simulink model "prob1"  (R2020a)
settings: Solver=VariableStepAuto  StartTime=0.0  StopTime=50  RelTol=1e-3
model workspace (MAT data in the model file):
  b = Simulink.Parameter
  b.Value = 50
  b.DataType = 'auto'
  b.Dimensions = [1 1]
  k1 = Simulink.Parameter
  k1.Value = 50
  k1.DataType = 'auto'
  k1.Dimensions = [1 1]
  k12 = Simulink.Parameter
  k12.Value = 10
  k12.DataType = 'auto'
  k12.Dimensions = [1 1]
  m1 = Simulink.Parameter
  m1.Value = 100
  m1.DataType = 'auto'
  m1.Dimensions = [1 1]
  m2 = Simulink.Parameter
  m2.Value = 45
  m2.DataType = 'auto'
  m2.Dimensions = [1 1]
  pi = Simulink.Parameter
  pi.Value = 3.14159
  pi.DataType = 'auto'
  pi.Dimensions = [1 1]
settings Model: Creator=akhil singh  LastModifiedBy=akhil singh

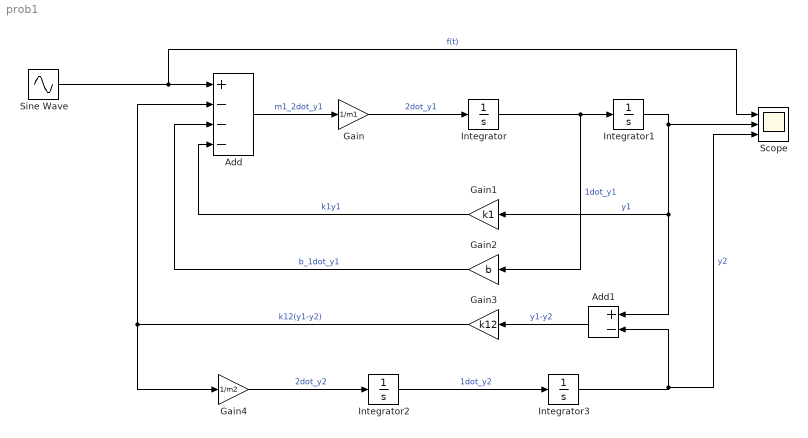
== system prob1 ==
  Add : Sum  Inputs=+---
  Add1 : Sum  Inputs=+-
  Gain : Gain  Gain=1/m1
  Gain1 : Gain  Gain=k1
  Gain2 : Gain  Gain=b
  Gain3 : Gain  Gain=k12
  Gain4 : Gain  Gain=1/m2
  Integrator : Integrator  InitialCondition=1
  Integrator1 : Integrator
  Integrator2 : Integrator
  Integrator3 : Integrator
  Scope : Scope  NumInputPorts=3
  Sine Wave : Sin  Amplitude=10  Frequency=10*2*pi  SampleTime=0
  wires:
  Sine Wave/1 -> Scope/1, Add/1  "f(t)"
  Add/1 -> Gain/1  "m1_2dot_y1"
  Integrator/1 -> Gain2/1, Integrator1/1  "1dot_y1"
  Gain/1 -> Integrator/1  "2dot_y1"
  Integrator1/1 -> Add1/1, Gain1/1, Scope/2  "y1"
  Gain1/1 -> Add/4  "k1y1"
  Gain2/1 -> Add/3  "b_1dot_y1"
  Add1/1 -> Gain3/1  "y1-y2"
  Gain3/1 -> Gain4/1, Add/2  "k12(y1-y2)"
  Gain4/1 -> Integrator2/1  "2dot_y2"
  Integrator2/1 -> Integrator3/1  "1dot_y2"
  Integrator3/1 -> Scope/3, Add1/2  "y2"
